simulink model "Modulation_cosim"  (Simulink 7.0)
settings: Solver=FixedStepDiscrete  StartTime=0.0  StopTime=15.0  RelTol=1e-3
undefined symbols (not defined in the file or in its folder): image, port_label
libraries: aldec_ahdl x3
settings Model: Creator=arekg  LastModifiedBy=arekg
settings DataIOCC: SignalLoggingName=sigsOut
settings OptimizationCC: InlineInvariantSignals=on
settings DebuggingCC: SaveWithParameterizedLinksMsg=none  SignalResolutionControl=TryResolveAllWithWarning  SolverPrmCheckMsg=none  MultiTaskDSMMsg=warning  MultiTaskCondExecSysMsg=none
settings HardwareCC: TargetUnknown=on
settings RTWCC: IncludeERTFirstTime=on
settings GRTTargetCC: TargetFcnLib=ansi_tfl_tmw.mat  ModelReferenceCompliant=off  MatFileLogging=off

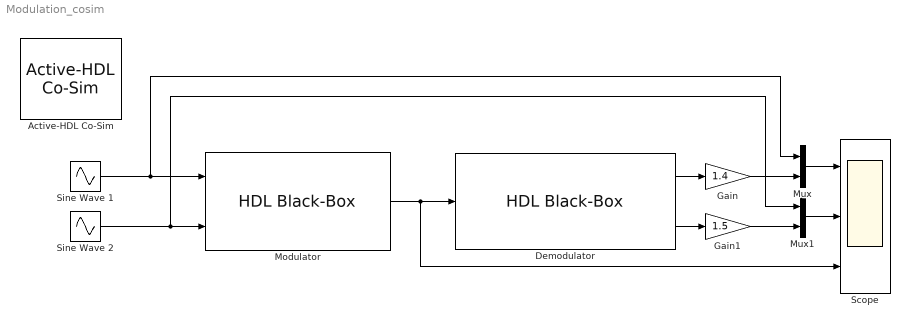
== system Modulation_cosim ==
  Active-HDL Co-Sim : aldec_ahdl/Active-HDL Co-Sim  Tag=Active-HDL_Co-Sim_close  hdl_period=1/40  hdl_tscale=sec  sys_period=[1/20, 0]  sys_tscale=As In Simulator  wav_fn=mlab_cosim  wav_settings=[0,0,0,0,0,0,0,0]  dbg=off  auto_start=off  gen_tb=[0,0,0]  batch_sim=off  tb_fn=mlab_post_tb.log  metavalue_map=[0,0]  sim_resolution=[1,0,0]  active_page=4  aws_en=off  ahdl_en=off  blk_ver=9.3.RTM  macro_en=[1,0,1]  macro_path=prepare_project.do  mfun_text=check_mfiles
  Demodulator : aldec_ahdl/HDL Black-Box  module_m=top_demodulator  ports_cfg={clk,3,1,0,0,Inherited,8,0,0,1,0,0}{reset,5,1,0,0,Inherited,8,0,0,1,0,0}{In1,0,31,0,24,Inherited,0,0,0,0,0,0}{envelope,1,21,0,5,clk,0,0,0,0,0,0}{carrier,1,21,0,5,clk,0,0,0,0,0,0}  clocks={0,2,0,0.5000,0}  stims={1,1 0ms 0 50ms}  hdl_src=c:\My_Designs\Samples_73\Simulink_modulation\Demodulator\src\fir_32.vhd;c:\My_Designs\Samples_73\Simulink_modulation\Demodulator\src\abs.vhd;c:\My_Designs\Samples_73\Simulink_modulation\Demodulator\src\sign.vhd;c:\My_Designs\Samples_73\Simulink_modulation\Demodulator\compile\top_demodulator.vhd  block_mask=image(imread('HDLBlackBox.jpg'),'center'); disp('top_demodulator');port_label('input', 1, 'In1');port_label('output', 1, 'envelope');port_label('output', 2, 'carrier');  config=[1,2]  inp=[1, 0, 31, 24, 0, 0, 0]  out=[2, 0, 21, 5, 0, 0, 0, 0, 21, 5, 0, 0, 0]  sampling=[1,-1,2,2]  active_page={0}{80,0,35,1,65,2,70,3,70,4,60,5,60,6,50,7,35,8,35,9,119,10}{103,0,55,1,70,2,75,3,75,4,45,5,45,6,45,7,165,8,0,0,0,0}{165,0,130,1,190,2,190,3,0,0,0,0,0,0,0,0,0,0,0,0,0,0}{81,0,60,1,60,2,70,3,60,4,0,0,0,0,0,0,0,0,0,0,0,0}{83,0,70,1,80,2,50,3,50,4,0,0,0,0,0,0,0,0,0,0,0,0}{125,0,330,1,220,2,0,0,0,0,0,0,0,0,0,0,0,0,0,0,0,0}{95,0,95,1,70,2,50,3,80,4,35,5,35,6,65,7,150,8,0,0,0,0}{735,436}  param_val=0  clk_val=[2,0,0.5000]  ce_val=[0]  blk_ver=9.3.RTM  blk_conf=0  user_conv=0
  Gain : Gain  Gain=1.4  ParameterDataType=sfix(16)  ParameterScaling=2^0  OutDataType=sfix(16)  OutScaling=2^0
  Gain1 : Gain  Gain=1.5  ParameterDataType=sfix(16)  ParameterScaling=2^0  OutDataType=sfix(16)  OutScaling=2^0
  Modulator : aldec_ahdl/HDL Black-Box  module_m=mult  ports_cfg={Sin_wav1,0,16,0,9,Inherited,0,0,0,0,0,0}{Sin_wav2,0,16,0,15,Inherited,0,0,0,0,0,0}{Out1,1,31,0,24,2,0,0,0,0,0,0}  hdl_src=c:\My_Designs\Samples_73\Simulink_modulation\modulator\src\mult.vhd  block_mask=image(imread('HDLBlackBox.jpg'),'center'); disp('mult');port_label('input', 1, 'Sin_wav1');port_label('input', 2, 'Sin_wav2');port_label('output', 1, 'Out1');  config=[2,1]  inp=[2, 0, 16, 9, 0, 0, 0, 0, 16, 15, 0, 0, 0]  out=[1, 0, 31, 24, 0, 0, 0]  sampling=[1,-1,-1,2]  active_page={0}{80,0,35,1,65,2,70,3,70,4,60,5,60,6,50,7,35,8,35,9,119,10}{103,0,55,1,70,2,75,3,75,4,45,5,45,6,45,7,165,8,0,0,0,0}{165,0,130,1,190,2,190,3,0,0,0,0,0,0,0,0,0,0,0,0,0,0}{81,0,60,1,60,2,70,3,60,4,0,0,0,0,0,0,0,0,0,0,0,0}{83,0,70,1,80,2,50,3,50,4,0,0,0,0,0,0,0,0,0,0,0,0}{125,0,330,1,220,2,0,0,0,0,0,0,0,0,0,0,0,0,0,0,0,0}{95,0,95,1,70,2,50,3,80,4,35,5,35,6,65,7,150,8,0,0,0,0}{735,436}  param_val=0  clk_val=[0]  ce_val=[0]  blk_ver=9.3.RTM  blk_conf=0  user_conv=0
  Mux : Mux  Inputs=2
  Mux1 : Mux  Inputs=2
  Scope : Scope  NumInputPorts=3
      settings: TimeRange=15  YMin=0~-1.5~-40  YMax=40~1.5~40
  Sine Wave 1 : Sin  Amplitude=18  Bias=20  Frequency=0.2*(2*pi)  Phase=pi/1.3  SampleTime=1/20
  Sine Wave 2 : Sin  Amplitude=0.9  Frequency=1.18*(2*pi)  Phase=pi  SampleTime=1/20
  wires:
  Sine Wave 1/1 -> Modulator/1, Mux/1
  Sine Wave 2/1 -> Modulator/2, Mux1/1
  Modulator/1 -> Demodulator/1, Scope/3
  Mux/1 -> Scope/1
  Demodulator/1 -> Gain/1
  Gain/1 -> Mux/2
  Mux1/1 -> Scope/2
  Demodulator/2 -> Gain1/1
  Gain1/1 -> Mux1/2
